simulink model "Concatenate_TestGen10"  (R2017b)
settings: Solver=FixedStepDiscrete  StartTime=0.0  StopTime=10.0  RelTol=1e-3
settings Model: Creator=ktrinh  LastModifiedBy=ktrinh
settings DebuggingCC: ParameterOverflowMsg=none

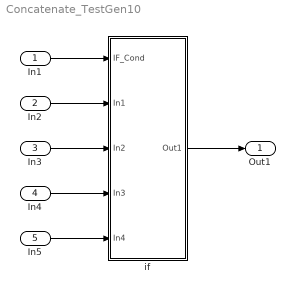
== system Concatenate_TestGen10 ==
  In1 : Inport
  In2 : Inport  Port=2
  In3 : Inport  Port=3
  In4 : Inport  Port=4
  In5 : Inport  Port=5
  if : Subsystem  AncestorBlock=Block_TestLib/if
  Out1 : Outport
  wires:
  In1/1 -> if/1(IF_Cond)
  In2/1 -> if/2(In1)
  In3/1 -> if/3(In2)
  In4/1 -> if/4(In3)
  In5/1 -> if/5(In4)
  if/1(Out1) -> Out1/1

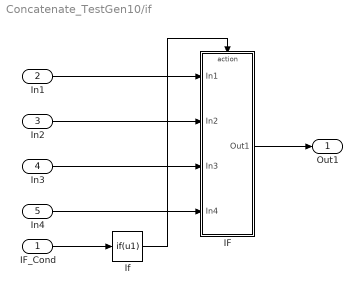
== system Concatenate_TestGen10/if ==
  IF_Cond : Inport  OutDataTypeStr=boolean
  In1 : Inport  Port=2
  In2 : Inport  Port=3
  In3 : Inport  Port=4
  In4 : Inport  Port=5
  IF : Subsystem  TreatAsAtomicUnit=on
  If : If  IfExpression=u1  ShowElse=off
  Out1 : Outport
  wires:
  If/1 -> IF/Action
  In1/1 -> IF/1(In1)
  In2/1 -> IF/2(In2)
  In3/1 -> IF/3(In3)
  In4/1 -> IF/4(In4)
  IF_Cond/1 -> If/1
  IF/1(Out1) -> Out1/1

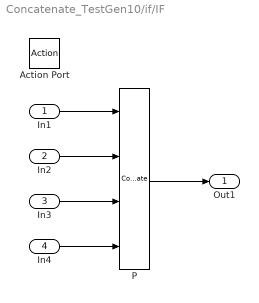
== system Concatenate_TestGen10/if/IF ==
  In1 : Inport  PortDimensions=[1 3]
  In2 : Inport  Port=2  PortDimensions=[1 3]
  In3 : Inport  Port=3  PortDimensions=[1 3]
  In4 : Inport  Port=4  PortDimensions=[1 3]
  Action Port : ActionPort  ActionType=then
  P : Concatenate  NumInputs=4
  Out1 : Outport
  wires:
  In1/1 -> P/1
  In2/1 -> P/2
  In3/1 -> P/3
  In4/1 -> P/4
  P/1 -> Out1/1
